simulink model "lab444"  (R2023b)
settings: Solver=VariableStepAuto  StartTime=0.0  StopTime=stop_time  MaxStep=0.001  RelTol=1e-3
values from neighbouring files (symbols this model uses):
  A = 50    [lab4.m]
  Ax = 10    [lab4.m]
  B = 54.2    [lab4.m]
  kr = 1.3    [lab4.m]
  mianownik = M{2}    [lab4.m]
  T = 1/100    (= 0.01)    [lab4.m]
  w = 1    [lab4.m]
settings Model: Creator=pc  LastModifiedBy=pc

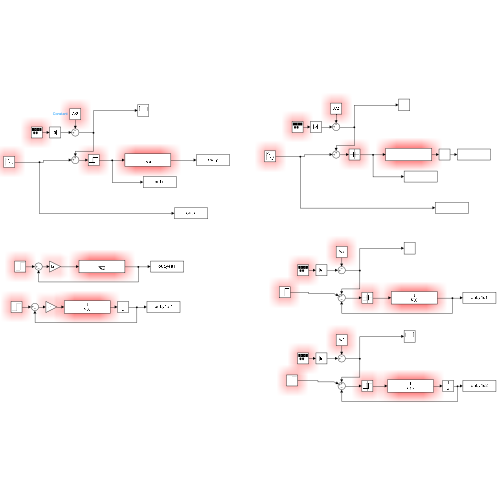
[thumbnail: Simulink's stored preview of the top-level diagram]
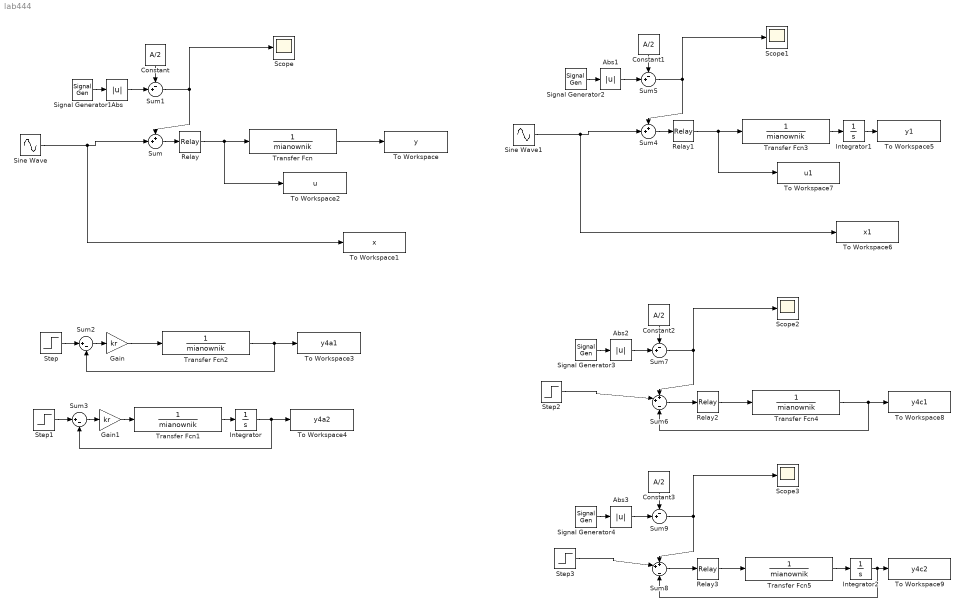
== system lab444 ==
  Abs{,1..3} (4 alike) : Abs  SaturateOnIntegerOverflow=off
  Constant{,1..3} (4 alike) : Constant  Value=A/2
  Gain : Gain  Gain=kr
  Gain1 : Gain  Gain=kr
  Integrator : Integrator
  Integrator1 : Integrator
  Integrator2 : Integrator
  Relay{,1..3} (4 alike) : Relay  OnSwitchValue=0  OffSwitchValue=0  OnOutputValue=B  OffOutputValue=-B
  Scope{,1..3} (4 alike) : Scope
  Signal Generator{1..4} (4 alike) : SignalGenerator  WaveForm=sawtooth  Amplitude=A  Frequency=1/T  Units=rad/sec
  Sine Wave : Sin  Amplitude=Ax  Frequency=0.1  SampleTime=0
  Sine Wave1 : Sin  Amplitude=Ax  Frequency=0.1  SampleTime=0
  Step{,1..3} (4 alike) : Step  Time=0  After=w  SampleTime=0
  Sum : Sum  Inputs=++|
  Sum{1,5,7,9} (4 alike) : Sum  Inputs=-+|
  Sum2 : Sum  Inputs=|+-
  Sum3 : Sum  Inputs=|+-
  Sum4 : Sum  Inputs=++|
  Sum6 : Sum  Inputs=++|-
  Sum8 : Sum  Inputs=++|-
  To Workspace : ToWorkspace  VariableName=y  SaveFormat=Timeseries  SampleTime=-1
  To Workspace1 : ToWorkspace  VariableName=x  SaveFormat=Timeseries  SampleTime=-1
  To Workspace2 : ToWorkspace  VariableName=u  SaveFormat=Timeseries  SampleTime=-1
  To Workspace3 : ToWorkspace  VariableName=y4a1  SaveFormat=Timeseries  SampleTime=-1
  To Workspace4 : ToWorkspace  VariableName=y4a2  SaveFormat=Timeseries  SampleTime=-1
  To Workspace5 : ToWorkspace  VariableName=y1  SaveFormat=Timeseries  SampleTime=-1
  To Workspace6 : ToWorkspace  VariableName=x1  SaveFormat=Timeseries  SampleTime=-1
  To Workspace7 : ToWorkspace  VariableName=u1  SaveFormat=Timeseries  SampleTime=-1
  To Workspace8 : ToWorkspace  VariableName=y4c1  SaveFormat=Timeseries  SampleTime=-1
  To Workspace9 : ToWorkspace  VariableName=y4c2  SaveFormat=Timeseries  SampleTime=-1
  Transfer Fcn{,1..5} (6 alike) : TransferFcn  Denominator=mianownik
  wires:
  Signal Generator1/1 -> Abs/1
  Sum/1 -> Relay/1
  Relay/1 -> To Workspace2/1, Transfer Fcn/1
  Abs/1 -> Sum1/2
  Sum1/1 -> Scope/1, Sum/1
  Constant/1 -> Sum1/1
  Sine Wave/1 -> To Workspace1/1, Sum/2
  Transfer Fcn/1 -> To Workspace/1
  Gain/1 -> Transfer Fcn2/1
  Step/1 -> Sum2/1
  Sum2/1 -> Gain/1
  Transfer Fcn2/1 -> Sum2/2, To Workspace3/1
  Sum3/1 -> Gain1/1
  Step1/1 -> Sum3/1
  Gain1/1 -> Transfer Fcn1/1
  Transfer Fcn1/1 -> Integrator/1
  Integrator/1 -> Sum3/2, To Workspace4/1
  Transfer Fcn3/1 -> Integrator1/1
  Sine Wave1/1 -> Sum4/2, To Workspace6/1
  Constant1/1 -> Sum5/1
  Sum5/1 -> Sum4/1, Scope1/1
  Abs1/1 -> Sum5/2
  Relay1/1 -> Transfer Fcn3/1, To Workspace7/1
  Sum4/1 -> Relay1/1
  Signal Generator2/1 -> Abs1/1
  Integrator1/1 -> To Workspace5/1
  Transfer Fcn4/1 -> Sum6/3, To Workspace8/1
  Sum7/1 -> Scope2/1, Sum6/1
  Step2/1 -> Sum6/2
  Constant2/1 -> Sum7/1
  Relay2/1 -> Transfer Fcn4/1
  Abs2/1 -> Sum7/2
  Sum6/1 -> Relay2/1
  Signal Generator3/1 -> Abs2/1
  Abs3/1 -> Sum9/2
  Signal Generator4/1 -> Abs3/1
  Sum8/1 -> Relay3/1
  Sum9/1 -> Scope3/1, Sum8/1
  Relay3/1 -> Transfer Fcn5/1
  Constant3/1 -> Sum9/1
  Step3/1 -> Sum8/2
  Transfer Fcn5/1 -> Integrator2/1
  Integrator2/1 -> Sum8/3, To Workspace9/1
